simulink model "P4_EV"  (R2023b)
settings: Solver=ode45  StartTime=0.0  StopTime=3600  MaxStep=5.0  RelTol=1e-3
undefined symbols (not defined in the file or in its folder): batData, carData, motorData, track_radius
libraries: slpidlib x1
settings Model: NumberOfSteps=100  Creator=Matt Cain  LastModifiedBy=Rehman Deen

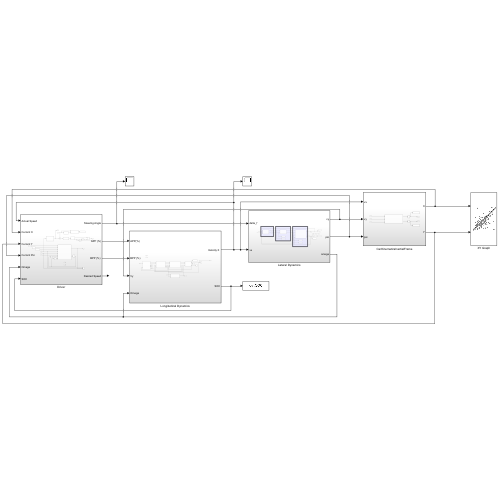
[thumbnail: Simulink's stored preview of the top-level diagram]
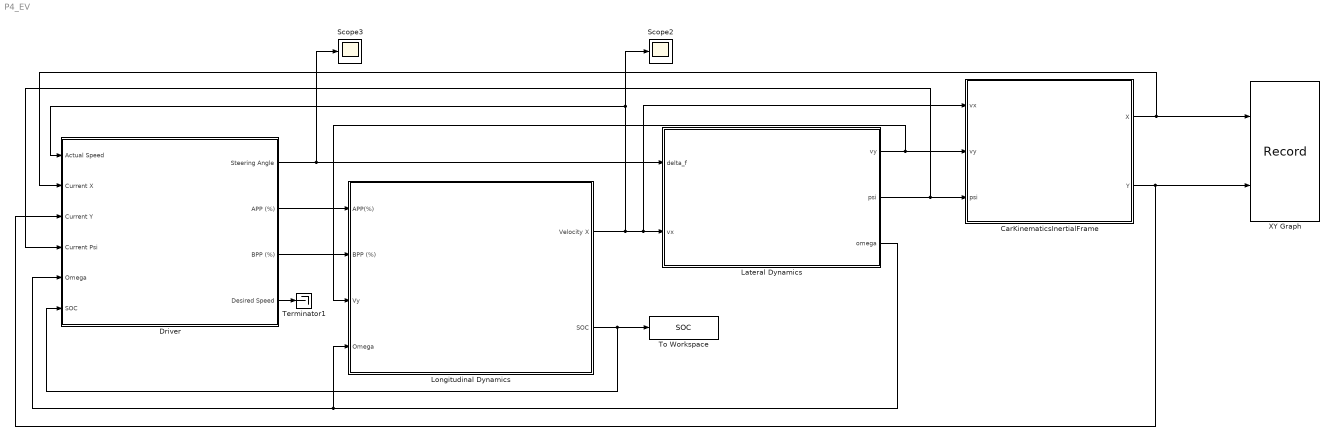
== system P4_EV ==
  CarKinematicsInertialFrame : Subsystem
  "Driver " : Subsystem
  Lateral Dynamics : Subsystem
  Longitudinal Dynamics : Subsystem
  Scope2 : Scope
  Scope3 : Scope
  Terminator1 : Terminator
  To Workspace : ToWorkspace  VariableName=SOC  SaveFormat=Timeseries  SampleTime=-1
  XY Graph : Record  FileSettingsInternal="{\"entries\":[{\"content\":{\"excelSettings\":{\"content\":{},\"type\":\"Streamout.ExcelSettings\"}},\"type\":\"Streamout.FileSettingStorage\",\"uuid\":\"\"}],\"packageUris\":[\"http:\\/\\/schema.mathworks.com\\/mf0\\/streamout_blocks\\/R2020a\"],\"version\":\"1.0\"}"  Layout=[1 1]  SignalsInternal="{\"entries\":[{\"content\":{\"signals\":[{\"content\":{\"blockPath\":[],\"dimensions\":[1],\"domain\":\"\",\"lineColor\":\"#fe330a\",\"port\":1,\"signalID\":8,\"signalName\":\"CarKinematicsInertialFrame1:1\"},\"type\":\"RecordBlkView.Signal\",\"uuid\":\"\"},{\"content\":{\"blockPath\":[],\"dimensions\":[1],\"domain\":\"\",\"lineColor\":\"#22b573\",\"port\":2,\"signalID\":11,\"signalName\":\"CarKinematicsInertialFrame1:2\"},\"type\":\"RecordBlkView.Signal\",\"uuid\":\"\"}]},\"type\":\"RecordBlkView.InputSignals\",\"uuid\":\"\"}],\"packageUris\":[\"http:\\/\\/schema.mathworks.com\\/mf0\\/streamout_blocks\\/R2020a\"],\"version\":\"1.0\"}"  VisualizationBindings="{\"xyplotplugin\":{\"info\":[{\"series\":[],\"subplotID\":1}]}}"  CompatibilityTag=XY  st=-1
  wires:
  CarKinematicsInertialFrame/1(X) -> XY Graph/1, "Driver "/2(Current X)
  CarKinematicsInertialFrame/2(Y) -> XY Graph/2, "Driver "/3(Current Y)
  Lateral Dynamics/1(vy) -> CarKinematicsInertialFrame/2(vy), Longitudinal Dynamics/3(Vy)
  Lateral Dynamics/2(psi) -> CarKinematicsInertialFrame/3(psi), "Driver "/4(Current Psi)
  Longitudinal Dynamics/1("Velocity X ") -> Lateral Dynamics/2(vx), CarKinematicsInertialFrame/1(vx), Scope2/1, "Driver "/1(Actual Speed)
  "Driver "/1(Steering Angle) -> Scope3/1, Lateral Dynamics/1(delta_f)
  "Driver "/2(APP (%)) -> Longitudinal Dynamics/1(APP(%))
  "Driver "/3("BPP (%) ") -> Longitudinal Dynamics/2(BPP (%))
  Lateral Dynamics/3(omega) -> "Driver "/5(Omega), Longitudinal Dynamics/4(Omega)
  Longitudinal Dynamics/2(SOC) -> To Workspace/1, "Driver "/6(SOC)
  "Driver "/4(Desired Speed) -> Terminator1/1

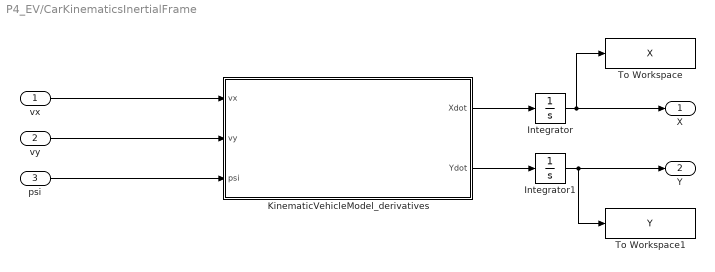
== system P4_EV/CarKinematicsInertialFrame ==
  vx : Inport
  vy : Inport  Port=2
  psi : Inport  Port=3
  Integrator : Integrator  InitialCondition=carData.init.X0
  Integrator1 : Integrator  InitialCondition=carData.init.Y0
  KinematicVehicleModel_derivatives : MATLAB Function  TreatAsAtomicUnit=on  mask{obj=carData}
      mask prompts: obj "obj structure"
  To Workspace : ToWorkspace  VariableName=X  SaveFormat=Structure With Time  SampleTime=-1
  To Workspace1 : ToWorkspace  VariableName=Y  SaveFormat=Structure With Time  SampleTime=-1
  X : Outport
  Y : Outport  Port=2
  wires:
  KinematicVehicleModel_derivatives/1(Xdot) -> Integrator/1
  KinematicVehicleModel_derivatives/2(Ydot) -> Integrator1/1
  Integrator/1 -> To Workspace/1, X/1
  Integrator1/1 -> To Workspace1/1, Y/1
  vx/1 -> KinematicVehicleModel_derivatives/1(vx)
  vy/1 -> KinematicVehicleModel_derivatives/2(vy)
  psi/1 -> KinematicVehicleModel_derivatives/3(psi)

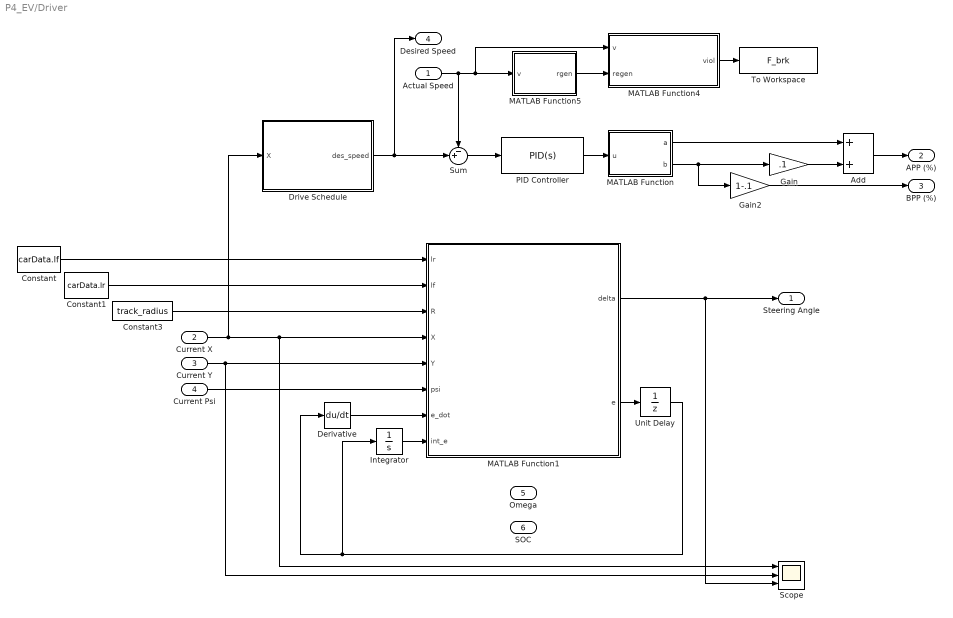
== system P4_EV/Driver  ==
  Actual Speed : Inport
  Current X : Inport  Port=2
  Current Y : Inport  Port=3
  Current Psi : Inport  Port=4
  Omega : Inport  Port=5
  SOC : Inport  Port=6
  Add : Sum
  Constant : Constant  Value=carData.lf
  Constant1 : Constant  Value=carData.lr
  Constant3 : Constant  Value=track_radius
  Derivative : Derivative
  Drive Schedule : MATLAB Function  TreatAsAtomicUnit=on
  Gain : Gain  Gain=.1
  Gain2 : Gain  Gain=1-.1
  Integrator : Integrator
  MATLAB Function : MATLAB Function  TreatAsAtomicUnit=on
  MATLAB Function1 : MATLAB Function  TreatAsAtomicUnit=on
  MATLAB Function4 : MATLAB Function  TreatAsAtomicUnit=on
  MATLAB Function5 : MATLAB Function  TreatAsAtomicUnit=on
  PID Controller : slpidlib/PID Controller  Controller=PID  Form=Parallel  TimeDomain=Continuous-time  UseExternalTs=off  SampleTime=-1  IntegratorMethod=Forward Euler  FilterMethod=Forward Euler  ControllerParametersSource=internal  P=.5  I=0  UseKiTs=off  D=0  N=100  UseFilter=on  TunerSelectOption=Transfer Function Based (PID Tuner App)  InitialConditionSource=internal  InitialConditionForIntegrator=0  InitialConditionForFilter=0  DifferentiatorICPrevScaledInput=0  ExternalReset=none  TrackingMode=off  Kt=1  LimitOutput=on  SatLimitsSource=internal  UpperSaturationLimit=1  LowerSaturationLimit=-1  LinearizeAsGain=off  AntiWindupMode=none  Kb=1  LimitIntegrator=off  UpperIntegratorSaturationLimit=inf  LowerIntegratorSaturationLimit=-inf  POutMin=[]  POutMax=[]  IOutMin=[]  IOutMax=[]  DOutMin=[]  DOutMax=[]  NOutMin=[]  NOutMax=[]  SumOutMin=[]  SumOutMax=[]  SaturationOutMin=[]  SaturationOutMax=[]  PParamMin=[]  PParamMax=[]  IParamMin=[]  IParamMax=[]  DParamMin=[]  DParamMax=[]  NParamMin=[]  NParamMax=[]  KbParamMin=[]  KbParamMax=[]  KtParamMin=[]  KtParamMax=[]  KbOutMin=[]  KbOutMax=[]  KtOutMin=[]  KtOutMax=[]  IntegratorOutMin=[]  IntegratorOutMax=[]  FilterOutMin=[]  FilterOutMax=[]  SumI1OutMin=[]  SumI1OutMax=[]  SumI2OutMin=[]  SumI2OutMax=[]  SumI3OutMin=[]  SumI3OutMax=[]  SumI4OutMin=[]  SumI4OutMax=[]  SumDOutMin=[]  SumDOutMax=[]  DifferentiatorOutMin=[]  DifferentiatorOutMax=[]  FilterDiffOutCoefMin=[]  FilterDiffOutCoefMax=[]  ReciprocalOutMin=[]  ReciprocalOutMax=[]  SumDenOutMin=[]  SumDenOutMax=[]  SumNumOutMin=[]  SumNumOutMax=[]  DivideOutMin=[]  DivideOutMax=[]  UdiffTsProdOutMin=[]  UdiffTsProdOutMax=[]  NTsProdOutMin=[]  NTsProdOutMax=[]  UintegralTsProdOutMin=[]  UintegralTsProdOutMax=[]  UngainTsProdOutMin=[]  UngainTsProdOutMax=[]  ClampingZeroOutDataTypeStr=Inherit: Inherit via back propagation  ClampingZeroOutMin=[]  ClampingZeroOutMax=[]  FilterDenConstantOutDataTypeStr=Inherit: Inherit via back propagation  FilterDenConstantOutMin=[]  FilterDenConstantOutMax=[]  PCopyOutDataTypeStr=Inherit: Inherit via back propagation  PCopyOutMin=[]  PCopyOutMax=[]  NCopyOutDataTypeStr=Inherit: Inherit via back propagation  NCopyOutMin=[]  NCopyOutMax=[]  IntegratorContinuousStateAttributes=''  IntegratorStateMustResolveToSignalObject=off  IntegratorRTWStateStorageClass=Auto  FilterContinuousStateAttributes=''  FilterStateMustResolveToSignalObject=off  FilterRTWStateStorageClass=Auto  ParallelPVariant=InternalParameters  IdealPVariant=Disabled  IVariant=InternalParameters  DVariant=InternalParameters  IntegratorVariant=Continuous  SatVariant=Enabled  AWVariant=Passthrough  PCopyVariant=Disabled  TRVariant=Disabled  FdbkBlocksVariant=Forward  IdealPFdbkVariant=Disabled  SatFdbkVariant=Disabled  DerivativeFilterVariant=ContFilter  NVariant=InternalParameters  NCopyVariant=Disabled  FilterICVariant=InternalICsFilter  IntegratorICVariant=InternalICs  ExternalResetVariant=Disabled  TRSumVariant=Passthrough  SumFdbkVariant=Disabled  SumVariant=Sum_PID  TsampFilterVariant=InternalTs  TsampNgainVariant=Passthrough  TsampIntegralVariant=Disabled_SignalSpec  ExternalSaturationOutDataTypeStr=Inherit: Same as second input
  Scope : Scope  NumInputPorts=3
  Sum : Sum  Inputs=-+|
  To Workspace : ToWorkspace  VariableName=F_brk  SaveFormat=Timeseries  SampleTime=-1
  Unit Delay : UnitDelay  SampleTime=-1  HasFrameUpgradeWarning=on
  Steering Angle : Outport
  APP (%) : Outport  Port=2
  "BPP (%) " : Outport  Port=3
  Desired Speed : Outport  Port=4
  wires:
  Actual Speed/1 -> MATLAB Function5/1(v), MATLAB Function4/1(v), Sum/1
  Sum/1 -> PID Controller/1
  PID Controller/1 -> MATLAB Function/1(u)
  Gain/1 -> Add/2
  Gain2/1 -> "BPP (%) "/1
  Add/1 -> APP (%)/1
  MATLAB Function/2(b) -> Gain/1, Gain2/1
  MATLAB Function/1(a) -> Add/1
  Drive Schedule/1(des_speed) -> Desired Speed/1, Sum/2
  MATLAB Function1/1(delta) -> Steering Angle/1, Scope/3
  Current Psi/1 -> MATLAB Function1/6(psi)
  Current Y/1 -> Scope/2, MATLAB Function1/5(Y)
  Constant3/1 -> MATLAB Function1/3(R)
  Constant1/1 -> MATLAB Function1/2(lf)
  MATLAB Function1/2(e) -> Unit Delay/1
  Constant/1 -> MATLAB Function1/1(lr)
  Integrator/1 -> MATLAB Function1/8(int_e)
  Current X/1 -> Scope/1, MATLAB Function1/4(X), Drive Schedule/1(X)
  Derivative/1 -> MATLAB Function1/7(e_dot)
  Unit Delay/1 -> Derivative/1, Integrator/1
  MATLAB Function5/1(rgen) -> MATLAB Function4/2(regen)
  MATLAB Function4/1(viol) -> To Workspace/1

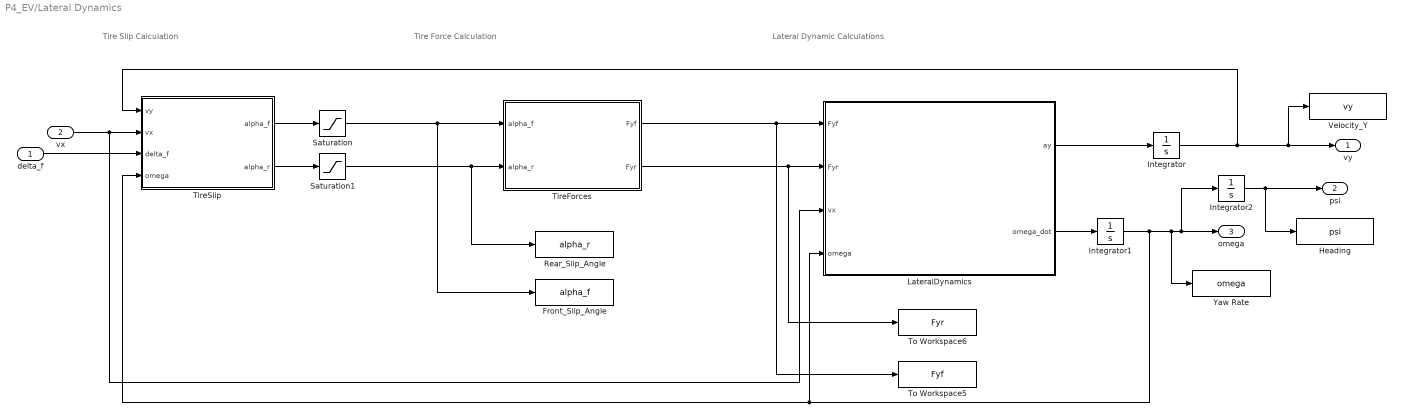
== system P4_EV/Lateral Dynamics ==
  note: Tire Slip Calculation
  note: Tire Force Calculation
  note: Lateral Dynamic Calculations
  delta_f : Inport
  vx : Inport  Port=2
  Front_Slip_Angle : ToWorkspace  VariableName=alpha_f  SaveFormat=Timeseries  SampleTime=-1
  Heading : ToWorkspace  VariableName=psi  SaveFormat=Timeseries  SampleTime=-1
  Integrator : Integrator  InitialCondition=carData.init.vy0
  Integrator1 : Integrator  InitialCondition=carData.init.omega0
  Integrator2 : Integrator  InitialCondition=carData.init.psi0
  LateralDynamics : MATLAB Function  TreatAsAtomicUnit=on  mask{obj=carData}
      mask prompts: obj "obj structure"
  Rear_Slip_Angle : ToWorkspace  VariableName=alpha_r  SaveFormat=Timeseries  SampleTime=-1
  Saturation : Saturate  UpperLimit=carData.maxAlpha  LowerLimit=-carData.maxAlpha
  Saturation1 : Saturate  UpperLimit=carData.maxAlpha  LowerLimit=-carData.maxAlpha
  TireForces : MATLAB Function  TreatAsAtomicUnit=on  mask{obj=carData}
      mask prompts: obj "obj structure"
  TireSlip : MATLAB Function  TreatAsAtomicUnit=on  mask{obj=carData}
      mask prompts: obj "obj structure"
  To Workspace5 : ToWorkspace  VariableName=Fyf  SaveFormat=Timeseries  SampleTime=-1
  To Workspace6 : ToWorkspace  VariableName=Fyr  SaveFormat=Timeseries  SampleTime=-1
  Velocity_Y : ToWorkspace  VariableName=vy  SaveFormat=Timeseries  SampleTime=-1
  Yaw Rate : ToWorkspace  VariableName=omega  SaveFormat=Timeseries  SampleTime=-1
  vy : Outport
  psi : Outport  Port=2
  omega : Outport  Port=3
  wires:
  LateralDynamics/1(ay) -> Integrator/1
  Integrator/1 -> vy/1, Velocity_Y/1, TireSlip/1(vy)
  LateralDynamics/2(omega_dot) -> Integrator1/1
  Integrator1/1 -> Integrator2/1, omega/1, Yaw Rate/1, LateralDynamics/4(omega), TireSlip/4(omega)
  TireSlip/1(alpha_f) -> Saturation/1
  TireSlip/2(alpha_r) -> Saturation1/1
  TireForces/1(Fyf) -> LateralDynamics/1(Fyf), To Workspace5/1
  TireForces/2(Fyr) -> LateralDynamics/2(Fyr), To Workspace6/1
  Saturation/1 -> TireForces/1(alpha_f), Front_Slip_Angle/1
  Saturation1/1 -> TireForces/2(alpha_r), Rear_Slip_Angle/1
  vx/1 -> TireSlip/2(vx), LateralDynamics/3(vx)
  delta_f/1 -> TireSlip/3(delta_f)
  Integrator2/1 -> Heading/1, psi/1

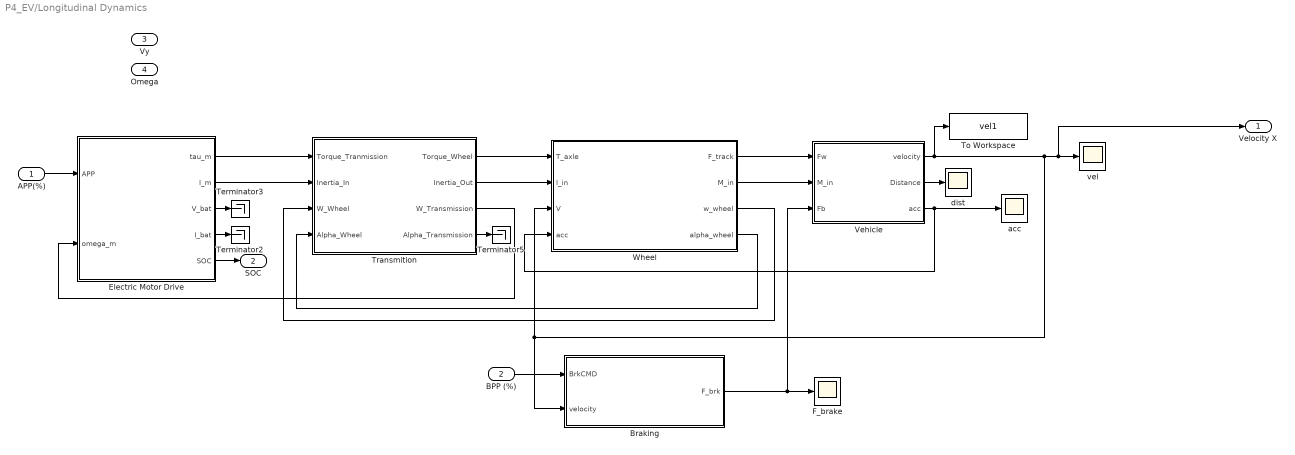
== system P4_EV/Longitudinal Dynamics ==
  APP(%) : Inport
  BPP (%) : Inport  Port=2
  Vy : Inport  Port=3
  Omega : Inport  Port=4
  Braking : Subsystem
  Electric Motor Drive : Subsystem
  F_brake : Scope
  Terminator2 : Terminator
  Terminator3 : Terminator
  Terminator5 : Terminator
  To Workspace : ToWorkspace  VariableName=vel1  SaveFormat=Timeseries  SampleTime=-1
  Transmition : Subsystem
  Vehicle : Subsystem
  "Wheel " : Subsystem
  acc : Scope
  dist : Scope
  vel : Scope
  "Velocity X " : Outport
  SOC : Outport  Port=2
  wires:
  "Wheel "/1(F_track) -> Vehicle/1("Fw ")
  Transmition/3(W_Transmission) -> Electric Motor Drive/2(omega_m)
  Electric Motor Drive/3(V_bat) -> Terminator3/1
  Vehicle/1("velocity ") -> vel/1, "Velocity X "/1, Braking/2("velocity "), "Wheel "/3(V), To Workspace/1
  Transmition/2(Inertia_Out) -> "Wheel "/2(I_in)
  Vehicle/3(acc) -> acc/1, "Wheel "/4(acc)
  Braking/1("F_brk ") -> F_brake/1, Vehicle/3("Fb ")
  Electric Motor Drive/2(I_m) -> Transmition/2(Inertia_In)
  Vehicle/2("Distance ") -> dist/1
  Electric Motor Drive/4(I_bat) -> Terminator2/1
  "Wheel "/2(M_in) -> Vehicle/2("M_in ")
  Electric Motor Drive/5(SOC) -> SOC/1
  Transmition/4(Alpha_Transmission) -> Terminator5/1
  Transmition/1(Torque_Wheel) -> "Wheel "/1(T_axle)
  "Wheel "/3(w_wheel) -> Transmition/3(W_Wheel)
  "Wheel "/4(alpha_wheel) -> Transmition/4(Alpha_Wheel)
  Electric Motor Drive/1(tau_m) -> Transmition/1(Torque_Tranmission)
  APP(%)/1 -> Electric Motor Drive/1(APP)
  BPP (%)/1 -> Braking/1("BrkCMD ")

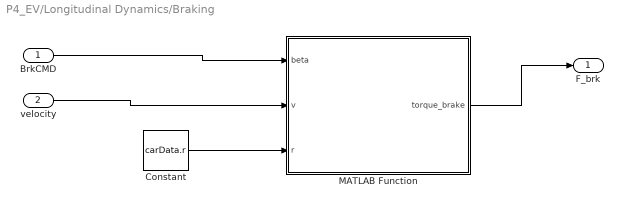
== system P4_EV/Longitudinal Dynamics/Braking ==
  "BrkCMD " : Inport
  "velocity " : Inport  Port=2
  Constant : Constant  Value=carData.r
  MATLAB Function : MATLAB Function  TreatAsAtomicUnit=on
  "F_brk " : Outport  VectorParamsAs1DForOutWhenUnconnected=off
  wires:
  "BrkCMD "/1 -> MATLAB Function/1(beta)
  MATLAB Function/1(torque_brake) -> "F_brk "/1
  "velocity "/1 -> MATLAB Function/2(v)
  Constant/1 -> MATLAB Function/3(r)

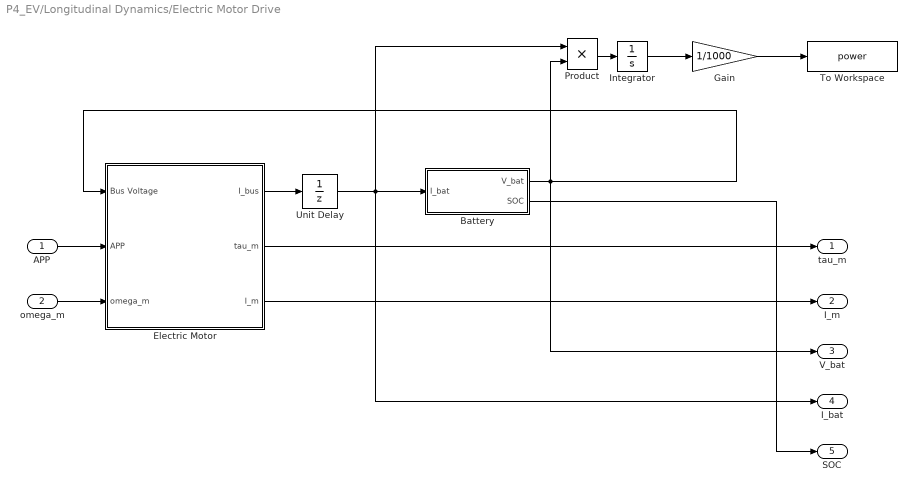
== system P4_EV/Longitudinal Dynamics/Electric Motor Drive ==
  APP : Inport
  omega_m : Inport  Port=2
  Battery : Subsystem
  Electric Motor : Subsystem
  Gain : Gain  Gain=1/1000
  Integrator : Integrator
  Product : Product
  To Workspace : ToWorkspace  VariableName=power  SaveFormat=Timeseries  SampleTime=-1
  Unit Delay : UnitDelay  SampleTime=-1  HasFrameUpgradeWarning=on
  tau_m : Outport
  I_m : Outport  Port=2
  V_bat : Outport  Port=3
  I_bat : Outport  Port=4
  SOC : Outport  Port=5
  wires:
  APP/1 -> Electric Motor/2(APP)
  omega_m/1 -> Electric Motor/3(omega_m)
  Electric Motor/1(I_bus) -> Unit Delay/1
  Battery/1(V_bat) -> Product/2, V_bat/1, Electric Motor/1(Bus Voltage)
  Battery/2(SOC) -> SOC/1
  Electric Motor/3(I_m) -> I_m/1
  Electric Motor/2(tau_m) -> tau_m/1
  Unit Delay/1 -> Product/1, I_bat/1, Battery/1(I_bat)
  Product/1 -> Integrator/1
  Integrator/1 -> Gain/1
  Gain/1 -> To Workspace/1

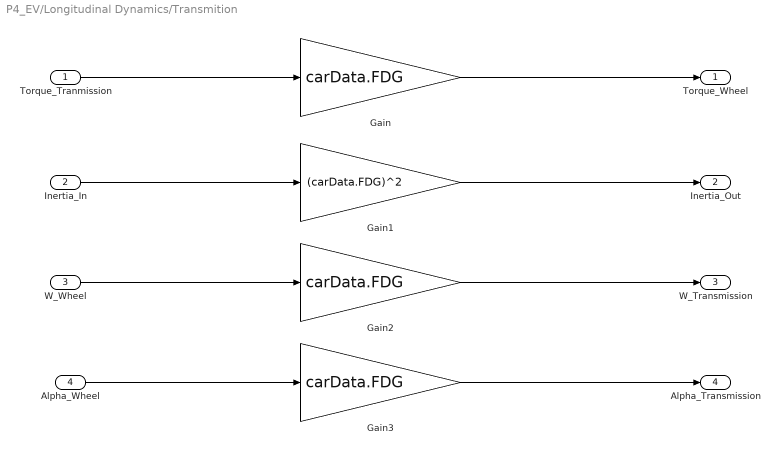
== system P4_EV/Longitudinal Dynamics/Transmition ==
  Torque_Tranmission : Inport
  Inertia_In : Inport  Port=2
  W_Wheel : Inport  Port=3
  Alpha_Wheel : Inport  Port=4
  Gain : Gain  Gain=carData.FDG
  Gain1 : Gain  Gain=(carData.FDG)^2
  Gain2 : Gain  Gain=carData.FDG
  Gain3 : Gain  Gain=carData.FDG
  Torque_Wheel : Outport
  Inertia_Out : Outport  Port=2
  W_Transmission : Outport  Port=3
  Alpha_Transmission : Outport  Port=4
  wires:
  Torque_Tranmission/1 -> Gain/1
  Inertia_In/1 -> Gain1/1
  W_Wheel/1 -> Gain2/1
  Alpha_Wheel/1 -> Gain3/1
  Gain/1 -> Torque_Wheel/1
  Gain1/1 -> Inertia_Out/1
  Gain2/1 -> W_Transmission/1
  Gain3/1 -> Alpha_Transmission/1

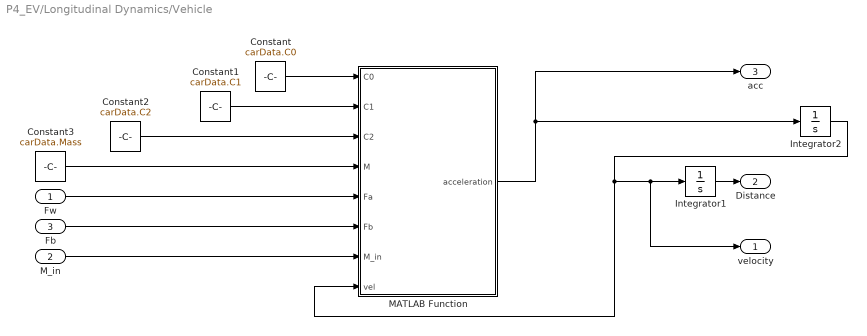
== system P4_EV/Longitudinal Dynamics/Vehicle ==
  "Fw " : Inport
  "M_in " : Inport  Port=2
  "Fb " : Inport  Port=3
  Constant : Constant  Value=carData.C0
  Constant1 : Constant  Value=carData.C1
  Constant2 : Constant  Value=carData.C2
  Constant3 : Constant  Value=carData.Mass
  Integrator1 : Integrator
  Integrator2 : Integrator  LimitOutput=on  LowerSaturationLimit=0
  MATLAB Function : MATLAB Function  TreatAsAtomicUnit=on
  "velocity " : Outport  VectorParamsAs1DForOutWhenUnconnected=off
  "Distance " : Outport  Port=2  VectorParamsAs1DForOutWhenUnconnected=off
  acc : Outport  Port=3
  wires:
  Constant1/1 -> MATLAB Function/2(C1)
  Constant/1 -> MATLAB Function/1(C0)
  Constant2/1 -> MATLAB Function/3(C2)
  Constant3/1 -> MATLAB Function/4(M)
  "Fw "/1 -> MATLAB Function/5(Fa)
  "Fb "/1 -> MATLAB Function/6(Fb)
  Integrator1/1 -> "Distance "/1
  "M_in "/1 -> MATLAB Function/7(M_in)
  MATLAB Function/1(acceleration) -> Integrator2/1, acc/1
  Integrator2/1 -> MATLAB Function/8(vel), "velocity "/1, Integrator1/1

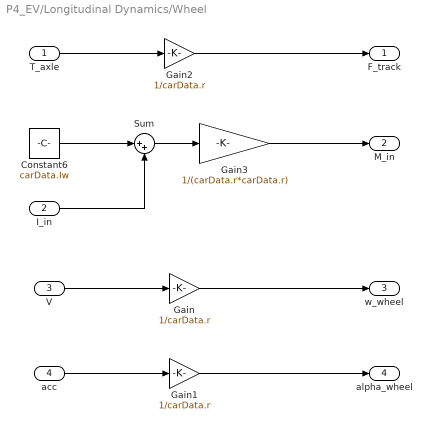
== system P4_EV/Longitudinal Dynamics/Wheel  ==
  T_axle : Inport
  I_in : Inport  Port=2
  V : Inport  Port=3
  acc : Inport  Port=4
  Constant6 : Constant  Value=carData.Iw
  Gain : Gain  Gain=1/carData.r
  Gain1 : Gain  Gain=1/carData.r
  Gain2 : Gain  Gain=1/carData.r
  Gain3 : Gain  Gain=1/(carData.r*carData.r)
  Sum : Sum  Inputs=|++
  F_track : Outport
  M_in : Outport  Port=2
  w_wheel : Outport  Port=3
  alpha_wheel : Outport  Port=4
  wires:
  Gain/1 -> w_wheel/1
  V/1 -> Gain/1
  acc/1 -> Gain1/1
  Gain1/1 -> alpha_wheel/1
  T_axle/1 -> Gain2/1
  Gain2/1 -> F_track/1
  Gain3/1 -> M_in/1
  Constant6/1 -> Sum/1
  I_in/1 -> Sum/2
  Sum/1 -> Gain3/1

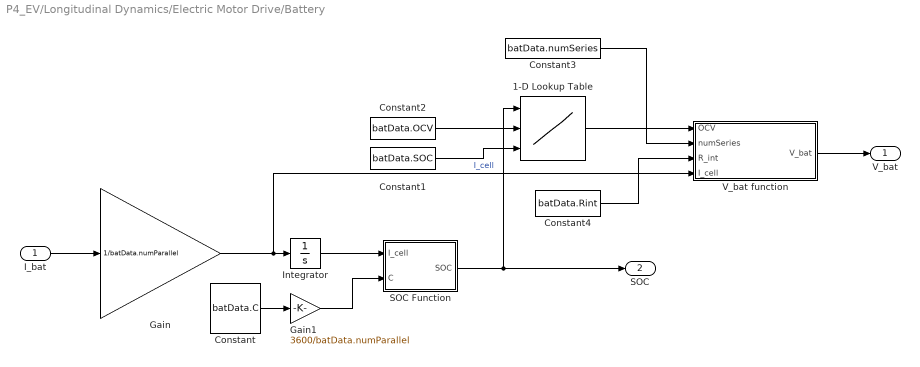
== system P4_EV/Longitudinal Dynamics/Electric Motor Drive/Battery ==
  I_bat : Inport
  1-D Lookup Table : Lookup_n-D  NumberOfTableDimensions=1  BreakpointsForDimension1Source=Input port  BreakpointsForDimension1=[-5:5]  TableSource=Input port  Table=tanh([-5:5])  InternalRulePriority=Speed  RndMeth=Simplest
      settings: InputPortMap=u0,p221,p5
  Constant : Constant  Value=batData.C
  Constant1 : Constant  Value=batData.SOC
  Constant2 : Constant  Value=batData.OCV
  Constant3 : Constant  Value=batData.numSeries
  Constant4 : Constant  Value=batData.Rint
  Gain : Gain  Gain=1/batData.numParallel
  Gain1 : Gain  Gain=3600/batData.numParallel
  Integrator : Integrator
  SOC Function : MATLAB Function  TreatAsAtomicUnit=on
  V_bat function : MATLAB Function  TreatAsAtomicUnit=on
  V_bat : Outport
  SOC : Outport  Port=2
  wires:
  I_bat/1 -> Gain/1
  Gain/1 -> V_bat function/4(I_cell), Integrator/1  "I_cell"
  Integrator/1 -> SOC Function/1(I_cell)
  Constant/1 -> Gain1/1
  SOC Function/1(SOC) -> 1-D Lookup Table/1, SOC/1
  Constant3/1 -> V_bat function/2(numSeries)
  V_bat function/1(V_bat) -> V_bat/1
  Constant4/1 -> V_bat function/3(R_int)
  Constant2/1 -> 1-D Lookup Table/2
  Constant1/1 -> 1-D Lookup Table/3
  1-D Lookup Table/1 -> V_bat function/1(OCV)
  Gain1/1 -> SOC Function/2(C)

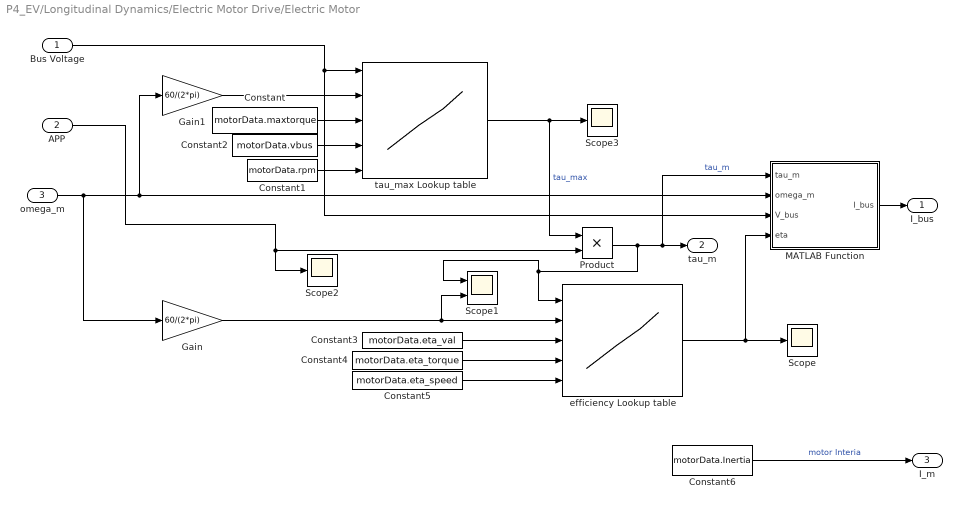
== system P4_EV/Longitudinal Dynamics/Electric Motor Drive/Electric Motor ==
  Bus Voltage : Inport
  APP : Inport  Port=2
  omega_m : Inport  Port=3
  Constant : Constant  Value=motorData.maxtorque
  Constant1 : Constant  Value=motorData.rpm
  Constant2 : Constant  Value=motorData.vbus
  Constant3 : Constant  Value=motorData.eta_val
  Constant4 : Constant  Value=motorData.eta_torque
  Constant5 : Constant  Value=motorData.eta_speed
  Constant6 : Constant  Value=motorData.Inertia
  Gain : Gain  Gain=60/(2*pi)
  Gain1 : Gain  Gain=60/(2*pi)
  MATLAB Function : MATLAB Function  TreatAsAtomicUnit=on
  Product : Product
  Scope : Scope
  Scope1 : Scope  NumInputPorts=2
  Scope2 : Scope
  Scope3 : Scope
  efficiency Lookup table : Lookup_n-D  BreakpointsForDimension1Source=Input port  BreakpointsForDimension1=[1:3]  BreakpointsForDimension2Source=Input port  BreakpointsForDimension2=[1:3]  BeginIndexSearchUsingPreviousIndexResult=on  TableSource=Input port  InternalRulePriority=Speed  RndMeth=Simplest
      settings: InputPortMap=u0,u1,p221,p5,p7
  tau_max Lookup table : Lookup_n-D  BreakpointsForDimension1Source=Input port  BreakpointsForDimension1=[1:3]  BreakpointsForDimension2Source=Input port  BreakpointsForDimension2=[1:3]  TableSource=Input port  InternalRulePriority=Speed  RndMeth=Simplest
      settings: InputPortMap=u0,u1,p221,p5,p7
  I_bus : Outport
  tau_m : Outport  Port=2
  I_m : Outport  Port=3
  wires:
  Constant/1 -> tau_max Lookup table/3
  Bus Voltage/1 -> tau_max Lookup table/1, MATLAB Function/3(V_bus)
  APP/1 -> Scope2/1, Product/2
  tau_max Lookup table/1 -> Product/1, Scope3/1  "tau_max"
  Product/1 -> efficiency Lookup table/1, Scope1/1, MATLAB Function/1(tau_m), tau_m/1  "tau_m"
  Constant3/1 -> efficiency Lookup table/3
  Constant4/1 -> efficiency Lookup table/4
  Constant5/1 -> efficiency Lookup table/5
  efficiency Lookup table/1 -> MATLAB Function/4(eta), Scope/1
  MATLAB Function/1(I_bus) -> I_bus/1
  Constant6/1 -> I_m/1  "motor Interia"
  Constant2/1 -> tau_max Lookup table/4
  Constant1/1 -> tau_max Lookup table/5
  omega_m/1 -> Gain/1, MATLAB Function/2(omega_m), Gain1/1
  Gain/1 -> Scope1/2, efficiency Lookup table/2
  Gain1/1 -> tau_max Lookup table/2

== matlab function P4_EV/Lateral Dynamics/TireSlip ==
  data: vy input size=1; vx input; delta_f input size=1; omega input; alpha_f output; obj parameter; alpha_r output
function [alpha_f, alpha_r] = fcn(vy,  vx, delta_f, omega, obj)


if abs(vx)> obj.vx_threshold1
      alpha_f = delta_f - (vy + omega * obj.lf) / vx;
      alpha_r = - (vy - omega * obj.lr) / vx;
else
      alpha_f = 0;
      alpha_r = 0;
end



end

== matlab function P4_EV/Driver /MATLAB Function ==
  data: u input; a output; b output
function [a,b] = fcn( u)

if u>0
    acc=u;
    brk=0;
elseif u<0
    acc=0;
    brk=-u;
else
    acc=0;
    brk=0;
end
a= acc;
b= brk;

== matlab function P4_EV/Longitudinal Dynamics/Electric Motor Drive/Battery/SOC Function ==
  data: I_cell input; C input; SOC output
function SOC= fcn(I_cell,C)

SOC = .8-I_cell/C;

== matlab function P4_EV/Longitudinal Dynamics/Electric Motor Drive/Battery/V_bat function ==
  data: OCV input; V_bat output; numSeries input; R_int input; I_cell input
function V_bat = fcn(OCV, numSeries, R_int, I_cell)

V_bat = numSeries * (OCV - R_int * I_cell);

== matlab function P4_EV/Longitudinal Dynamics/Electric Motor Drive/Electric Motor/MATLAB Function ==
  data: tau_m input; I_bus output; omega_m input; V_bus input; eta input
function I_bus = fcn(tau_m,omega_m,V_bus,eta)

% disp('tau_m');
% disp(tau_m);
% disp('omega');
% disp(omega_m);


Pm = tau_m * omega_m;

% disp('Pm');
% disp(Pm);
% disp('eta');
% disp(eta);
% disp('exp');
% disp(Pm/(abs(Pm)+.001));


Pe = Pm * (eta ^ complex(Pm/(abs(Pm)+.001)));
I_bus = real(Pe)/V_bus;

== matlab function P4_EV/Longitudinal Dynamics/Vehicle/MATLAB Function ==
  data: C0 input; acceleration output; C1 input; C2 input; M input; Fa input; Fb input; M_in input; vel input
function acceleration   = vehicle(C0,C1,C2,M,Fa,Fb,M_in, vel)

acceleration = (((Fa-Fb))-(C0+ C1*vel + C2*(vel)^2))/(M+M_in);

== matlab function P4_EV/Driver /MATLAB Function1 ==
  data: lr input; lf input; R input; X input; delta output; Y input; psi input; e_dot input; int_e input; e output
function [delta, e] = SimplestDriver(lr, lf, R, X, Y, psi, e_dot, int_e)

% Look Ahead Distance
l = 5;

% PID Coefficients
kp = .0016;
kd = 0;
ki = 0;
if X > 900
    theta = atan(200-Y/X-900);
    eta = l/R;
    psi_desired = psi+theta;
    e = psi - psi_desired;
    PID = kp*e + kd*e_dot + ki*int_e;
    delta = PID + (lr+lf)/R;
elseif X < 0
    theta = atan(200-Y/X - 900);
    eta = l/R;
    psi_desired = psi+theta;
    e = psi - psi_desired;
    PID = kp*e + kd*e_dot + ki*int_e;
    delta = PID + (lr+lf)/R;

else
    delta = 0;
    psi_desired = 0;
    e = psi-psi_desired;
    kp = .00049;
    kd = 0.0004/1000000;
    ki = 0.00000000009/100000000;
    if Y < 200
        l= 45;
        d = -Y;
        psi_desired = atan(d/l);
        e = psi_desired;
        PID = kp*e + kd*e_dot + ki*int_e;
        delta = PID;
    end
    if Y > 200
        l= -45;
        d = 400-Y;
        psi_desired = atan(d/l);
        e = psi_desired;
        PID = kp*e + kd*e_dot + ki*int_e;
        delta = PID;
    end
end

== matlab function P4_EV/Longitudinal Dynamics/Braking/MATLAB Function ==
  data: beta input; torque_brake output; v input; r input

function torque_brake = torque_brake(beta,v,r)
if beta == 0
    torque_brake = 0;
else
    torque_brake = beta * 10000 * (v / abs(v)+0.001) /r;
end

== matlab function P4_EV/Driver /Drive Schedule ==
  data: X input; des_speed output
function des_speed = fcn(X)

if X > 0  && X <15 || X < 900 && X > 885 % Slowing Down
    des_speed = 18; % 20

elseif X <= 885 && X >= 15 % Straights
    des_speed = 35; %36
else % Curves
    des_speed = 10; %10
end

== matlab function P4_EV/Driver /MATLAB Function4 ==
  data: v input; regen input; viol output
function viol = violfcn(v, regen)
    speed = (3600/1600)*v;
    if speed < 5
        regen_vio = 0;
        if regen == regen_vio
            viol = 0;
        else
            viol = 1;
        end

    elseif speed == 25
        regen_vio = 0.95;
        if regen == regen_vio
            viol = 0;
        else
            viol = 1;
        end

    elseif v > 25
        regen_vio = 0.95;
        if regen == regen_vio
            viol = 0;
        else
            viol = 1;
        end
    else
        regen_vio = ((0.95/20)*speed) - 0.2375;
        if regen == regen_vio
            viol = 0;
        else
            viol = 1;
        end
    end

== matlab function P4_EV/Driver /MATLAB Function5 ==
  data: v input; rgen output
function rgen = fcn(v)
if v <= 5
    rgen = 0;
  
elseif v > 5
    rgen = 0.0475 * (v-5);
    
else
    rgen = .95;
    
end

== matlab function P4_EV/CarKinematicsInertialFrame/KinematicVehicleModel_derivatives ==
  data: vx input; vy input; psi input size=1; Xdot output; Ydot output
function [Xdot, Ydot] = fcn(vx, vy, psi)
    temp = TF(psi) * [vx;vy]; 
    Xdot = temp(1);
    Ydot = temp(2);
  
end

function y = TF(psi)
    y = [cos(psi), -sin(psi); sin(psi), cos(psi)];
end

== matlab function P4_EV/Lateral Dynamics/LateralDynamics ==
  data: Fyf input; Fyr input size=1; vx input; omega input; ay output; obj parameter; omega_dot output
function [ay, omega_dot] = fcn(Fyf, Fyr, vx, omega, obj)

Fy = Fyf + Fyr;
ay = Fy / obj.Mass - omega * vx;
        
M  = Fyf * obj.lf - Fyr * obj.lr;        
omega_dot = M / obj.Inertia;        

end

== matlab function P4_EV/Lateral Dynamics/TireForces ==
  data: alpha_f input; alpha_r input; Fyf output; obj parameter; Fyr output
function [Fyf, Fyr] = fcn(alpha_f, alpha_r, obj)

Fyf = min(obj.Fyfmax,obj.Calpha_f * alpha_f);
Fyr = min(obj.Fyrmax, obj.Calpha_r * alpha_r);
end
